simulink model "SalientPolePMSM"  (R2020b)
settings: Solver=VariableStepAuto  StartTime=0  StopTime=1  MaxStep=1e-4  RelTol=1e-4
values from neighbouring files (symbols this model uses):
  Bgain = 1    [DataSalientPolePMSM-DESKTOP-IINSHMA.m]    (also in DataSalientPolePMSM.m)
  Gcc_1ord = 1/(s/bandwidth(Gcc) + 1)    [DataSalientPolePMSM-DESKTOP-IINSHMA.m]    (also in DataSalientPolePMSM.m)
  lamdVec = mot.Ld*idVec+mot.lammg    [DataSalientPolePMSM-DESKTOP-IINSHMA.m]    (also in DataSalientPolePMSM.m)
  lamqVec = mot.Lq*iqVec    [DataSalientPolePMSM-DESKTOP-IINSHMA.m]    (also in DataSalientPolePMSM.m)
  TAB0_abc = Tabc_AB0^-1    [DataSalientPolePMSM-DESKTOP-IINSHMA.m]    (also in DataSalientPolePMSM.m)
  Tabc_AB0 = 2/3.*[     1       -1/2       -1/2 ... (first row only)    [DataSalientPolePMSM-DESKTOP-IINSHMA.m]    (also in DataSalientPolePMSM.m)
  Talphabeta_abc = Tabc_alphabeta^(-1)    [DataSalientPolePMSM-DESKTOP-IINSHMA.m]    (also in DataSalientPolePMSM.m)
undefined symbols (not defined in the file or in its folder): DiscIntNeverNeededParam, dqpll, inv, kid, kpd, magnitude, meas, mot, Obs, PI, stconv
libraries: simulink x53, pid_lib x3, powerlib x2, eeBldcCommutationLogic x1, electricdrivelib x1
(part 6 of 7)

== system SalientPolePMSM/FOC2/INVERTER2/INVERTER power driver ==
  note: INVERTER:
      | (-Ubus/2  :  +Ubus/2)
  note: INPUTS:
  note: OUTPUTS:
  note: solo Tpwm/2 perchè
      | controllo tempo discreto
  duties : Inport
  uBus : Inport  Port=2
  iabc : Inport  Port=3
  Constant1 : Constant  Value=0.5
  Inverter non idealities : Subsystem  Commented=on
  Product : Product
  Subtract : Sum  Inputs=+-
  Transport Delay : TransportDelay  DelayTime=inv.Tpwm/2
  delay_aproximation : Subsystem  Commented=on
  uabc_n* : Outport
  uabc_n*nonideal : Outport  Port=2
  wires:
  iabc/1 -> Inverter non idealities/3(iabc)
  duties/1 -> Subtract/1
  Inverter non idealities/1(uabc_dist) -> uabc_n*nonideal/1
  Constant1/1 -> Subtract/2
  uBus/1 -> Inverter non idealities/2(uBus), Product/2
  Product/1 -> Inverter non idealities/1(uabc), Transport Delay/1  "uabc"
  Subtract/1 -> Product/1
  Transport Delay/1 -> uabc_n*/1

== system SalientPolePMSM/FOC2/INVERTER2/SVM algorithm ==
  note: INPUTS:
      | voltage references
      | Alpha Beta axes
  note: OUTPUT
  VABref : Inport  PortDimensions=2
  uBus : Inport  Port=2  PortDimensions=1
  Gain : Gain  Gain=1000
  MATLAB Function : MATLAB Function  Commented=on  TreatAsAtomicUnit=on  SystemSampleTime=inv.Ts
  MATLAB Function1 : MATLAB Function  TreatAsAtomicUnit=on  SystemSampleTime=inv.Ts
  MATLAB Function2 : MATLAB Function  TreatAsAtomicUnit=on  SystemSampleTime=inv.Ts
  MATLAB Function4 : MATLAB Function  Commented=on  TreatAsAtomicUnit=on  SystemSampleTime=inv.Ts
  Mux : Mux  Commented=on  Inputs=3
  Mux1 : Mux  Inputs=3
  Scope : Scope  Commented=on  NumInputPorts=3
  Scope1 : Scope  Commented=on  NumInputPorts=2
  Scope2 : Scope  NumInputPorts=2
  duties : Outport  PortDimensions=3
  wires:
  Mux/1 -> MATLAB Function/1(XYZ)
  MATLAB Function4/3(Z) -> Scope/3, Mux/3
  MATLAB Function4/2(Y) -> Scope/2, Mux/2
  MATLAB Function4/1(X) -> Scope/1, Mux/1
  MATLAB Function/2(duty) -> Scope1/1
  uBus/1 -> [UBUS]
  VABref/1 -> MATLAB Function4/1(VABref), Gain/1
  MATLAB Function/1(sector) -> Scope1/2
  MATLAB Function1/3(Z) -> Mux1/3
  MATLAB Function1/2(Y) -> Mux1/2
  MATLAB Function1/1(X) -> Mux1/1
  Gain/1 -> MATLAB Function1/1(VABref)
  Mux1/1 -> MATLAB Function2/1(XYZ)
  MATLAB Function2/2(duty) -> duties/1, Scope2/1
  MATLAB Function2/1(sector) -> Scope2/2

== system SalientPolePMSM/INVERTER/INVERTER power driver/Inverter non idealities ==
  note: Transport delay: it
      | simulate the PWM
      | delay
  note: This allows to calculate the distortion voltages
      | with respect to the star point of the motor.
      | In fact, the motor model is built considering the
      | star point of the motor! Each voltage distortion
      | has been calculated with respect to the central
      | point of the inverter.
  uabc : Inport  PortDimensions=3
  uBus : Inport  Port=2  PortDimensions=1
  iabc : Inport  Port=3  PortDimensions=3
  Add : Sum
  Add1 : Sum  Inputs=-++
  Add2 : Sum
  Add3 : Sum
  Add4 : Sum  Inputs=+-
  Constant : Constant  Value=0.5
  Constant1 : Constant  Value=inv.nid.Vdm
  Divide : Product  Inputs=*/
  Gain : Gain  Gain=2*inv.nid.Vdm
  Gain1 : Gain  Gain=inv.nid.Vcm
  Gain2 : Gain  Gain=inv.nid.ttot/inv.Ts
  Gain3 : Gain  Gain=-1/3
  Product : Product
  Sign : Signum
  Sum of Elements : Sum  Inputs=+
  Transport Delay : TransportDelay  DelayTime=inv.Tpwm/2
  uabc_dist : Outport  PortDimensions=3
  wires:
  Constant/1 -> Add/2
  uabc/1 -> Add4/1, Divide/1
  uBus/1 -> Divide/2, Gain2/1
  Divide/1 -> Add/1
  Add/1 -> Gain/1
  Gain/1 -> Add1/1
  Constant1/1 -> Add1/2
  Gain1/1 -> Add1/3
  Gain2/1 -> Product/2
  iabc/1 -> Sign/1
  Sign/1 -> Gain1/1, Product/1
  Add1/1 -> Add2/1
  Product/1 -> Add2/2  "u_dist_abc_n"
  Add2/1 -> Sum of Elements/1, Add3/1  "uabc_n_dist"
  Sum of Elements/1 -> Gain3/1
  Gain3/1 -> Add3/2  "u_on"
  Add3/1 -> Add4/2  "uabc_o_dist"
  Add4/1 -> Transport Delay/1
  Transport Delay/1 -> uabc_dist/1

== system SalientPolePMSM/INVERTER/INVERTER power driver/delay_aproximation ==
  uabc : Inport
  Demux2 : Demux  Outputs=3
  Mux : Mux  Inputs=3
  Transfer Fcn : TransferFcn  Denominator=[inv.tauD 1]
  Transfer Fcn1 : TransferFcn  Denominator=[inv.tauD 1]
  Transfer Fcn2 : TransferFcn  Denominator=[inv.tauD 1]
  uabc_n* : Outport
  wires:
  Demux2/3 -> Transfer Fcn2/1
  Transfer Fcn/1 -> Mux/1
  Transfer Fcn2/1 -> Mux/3
  Transfer Fcn1/1 -> Mux/2
  Demux2/1 -> Transfer Fcn/1
  Demux2/2 -> Transfer Fcn1/1
  uabc/1 -> Demux2/1
  Mux/1 -> uabc_n*/1

== system SalientPolePMSM/Synchronous motor1/electrical equations/Clarke + Park 2 ==
  note: INPUTS
  note: OUTPUT
  abc : Inport
  thme : Inport  Port=2
  Add2 : Sum
  Add3 : Sum  Inputs=-+
  Cos2 : Trigonometry  Operator=cos
  Demux1 : Demux  Outputs=3
  Demux2 : Demux  Outputs=3
  Gain1 : Gain  Gain=Tabc_AB0  Multiplication=Matrix(K*u) (u vector)
  Gain10 : Gain  Gain=-1/sqrt(3)
  Gain9 : Gain  Gain=2
  Mux1 : Mux  Inputs=2
  Mux2 : Mux  Inputs=3
  Product{,1..3} (4 alike) : Product
  Scope : Scope  NumInputPorts=2
  Sin2 : Trigonometry
  Sum5 : Sum  Inputs=++|
  Terminator : Terminator
  dq : Outport
  U_A : Outport  Port=2
  U_B : Outport  Port=3
  wires:
  Demux2/3 -> Terminator/1
  Product/1 -> Add2/1
  Product1/1 -> Add2/2
  Cos2/1 -> Product/2, Product3/1
  Demux2/1 -> [U_A], Product3/2, Product1/1
  thme/1 -> Cos2/1, Sin2/1
  Product3/1 -> Add3/2
  Product2/1 -> Add3/1
  Demux2/2 -> [U_B], Product2/1, Product/1
  Sin2/1 -> Product2/2, Product1/2
  Mux1/1 -> dq/1
  Add3/1 -> Mux1/2
  Add2/1 -> Mux1/1
  Sum5/1 -> Gain10/1
  Gain9/1 -> Sum5/2
  Demux1/2 -> Gain9/1
  Demux1/3 -> Mux2/3
  Demux1/1 -> Mux2/1, Sum5/1
  Gain10/1 -> Mux2/2
  abc/1 -> Gain1/1, Demux1/1
  Gain1/1 -> Scope/1, Demux2/1
  [U_A] -> U_A/1
  [U_B] -> U_B/1

== system SalientPolePMSM/Synchronous motor1/electrical equations/Clarke + Park 3 ==
  note: OUTPUT
  note: INPUTS
  abc : Inport
  thme : Inport  Port=2
  Add2 : Sum
  Add3 : Sum  Inputs=-+
  Cos2 : Trigonometry  Operator=cos
  Demux2 : Demux  Outputs=3
  Gain : Gain  Gain=Tabc_AB0  Multiplication=Matrix(K*u) (u vector)
  Mux1 : Mux  Inputs=2
  Product{,1..3} (4 alike) : Product
  Sin2 : Trigonometry
  Terminator : Terminator
  dq : Outport
  wires:
  Mux1/1 -> dq/1
  Sin2/1 -> Product1/2, Product2/2
  Demux2/2 -> Product3/2, Product1/1
  Product2/1 -> Add3/1
  Product3/1 -> Add3/2
  thme/1 -> Sin2/1, Cos2/1
  Demux2/1 -> Product2/1, Product/1
  Cos2/1 -> Product3/1, Product/2
  Product1/1 -> Add2/2
  Add3/1 -> Mux1/2
  Add2/1 -> Mux1/1
  Product/1 -> Add2/1
  Gain/1 -> Demux2/1  "AB0"
  Demux2/3 -> Terminator/1
  abc/1 -> Gain/1

== system SalientPolePMSM/Synchronous motor1/electrical equations/Subsystem2 ==
  note: INPUTS
  note: OUTPUT
  thme : Inport
  abc : Inport  Port=2
  Add2 : Sum
  Add3 : Sum  Inputs=-+
  Cos2 : Trigonometry  Operator=cos
  Demux2 : Demux  Outputs=3
  Demux3 : Demux  Outputs=3
  Gain : Gain  Gain=Tabc_AB0  Multiplication=Matrix(K*u) (u vector)
  Gain2 : Gain  Gain=2
  Gain3 : Gain  Gain=-1/sqrt(3)
  Mux1 : Mux  Inputs=2
  Mux2 : Mux  Inputs=3
  Product{,1..3,5} (5 alike) : Product
  Sin2 : Trigonometry
  Terminator : Terminator
  qd : Outport
  wires:
  Demux2/3 -> Terminator/1
  Product/1 -> Add2/1
  Product1/1 -> Add2/2
  Cos2/1 -> Product/2, Product3/1
  Demux2/1 -> Product1/1, Product3/2
  thme/1 -> Cos2/1, Sin2/1
  Product3/1 -> Add3/2
  Product2/1 -> Add3/1
  Demux2/2 -> Product2/1, Product/1
  Sin2/1 -> Product2/2, Product1/2
  Mux1/1 -> qd/1
  Mux2/1 -> ?  "AB0"
  Gain2/1 -> Product5/2
  ? -> Demux3/1
  Demux3/1 -> Mux2/1, Product5/1
  Product5/1 -> Gain3/1
  Demux3/2 -> Gain2/1
  Demux3/3 -> Mux2/3
  Gain3/1 -> Mux2/2
  abc/1 -> Gain/1
  Gain/1 -> Demux2/1
  Add2/1 -> Mux1/1
  Add3/1 -> Mux1/2

== system SalientPolePMSM/Synchronous motor1/electrical equations/Subsystem4 ==
  note: INPUTS
  note: OUTPUT
  thme : Inport
  abc : Inport  Port=2
  Add2 : Sum
  Add3 : Sum  Inputs=-+
  Cos2 : Trigonometry  Operator=cos
  Demux1 : Demux  Outputs=3
  Demux2 : Demux  Outputs=3
  Gain : Gain  Gain=2
  Gain1 : Gain  Gain=-1/sqrt(3)
  Mux : Mux  Inputs=3
  Mux1 : Mux  Inputs=2
  Product{,1..4} (5 alike) : Product
  Sin2 : Trigonometry
  Terminator : Terminator
  dq : Outport
  wires:
  Demux1/3 -> Mux/3
  Gain1/1 -> Mux/2
  Product4/1 -> Gain1/1
  Gain/1 -> Product4/2
  Demux1/2 -> Gain/1
  Demux1/1 -> Mux/1, Product4/1
  abc/1 -> Demux1/1
  Demux2/3 -> Terminator/1
  Mux/1 -> Demux2/1  "AB0"
  Product/1 -> Add2/1
  Add2/1 -> Mux1/1
  Add3/1 -> Mux1/2
  Product1/1 -> Add2/2
  Cos2/1 -> Product/2, Product3/1
  Demux2/1 -> Product1/1, Product3/2
  thme/1 -> Cos2/1, Sin2/1
  Product3/1 -> Add3/2
  Product2/1 -> Add3/1
  Demux2/2 -> Product2/1, Product/1
  Sin2/1 -> Product2/2, Product1/2
  Mux1/1 -> dq/1

== system SalientPolePMSM/Synchronous motor2/electrical equations/Subsystem1 ==
  note: OUTPUT
  note: INPUTS
  abc : Inport
  thme : Inport  Port=2
  Add2 : Sum
  Add3 : Sum  Inputs=-+
  Cos2 : Trigonometry  Operator=cos
  Demux2 : Demux  Outputs=3
  Gain : Gain  Gain=Tabc_AB0  Multiplication=Matrix(K*u) (u vector)
  Mux1 : Mux  Inputs=2
  Product{,1..3} (4 alike) : Product
  Scope : Scope  NumInputPorts=2
  Sin2 : Trigonometry
  Terminator : Terminator
  dq : Outport
  wires:
  Mux1/1 -> dq/1
  Sin2/1 -> Product1/2, Product2/2
  Demux2/2 -> Product3/2, Product1/1
  Product2/1 -> Add3/1
  Product3/1 -> Add3/2
  thme/1 -> Sin2/1, Cos2/1
  Demux2/1 -> Product2/1, Product/1
  Cos2/1 -> Product3/1, Product/2
  Product1/1 -> Add2/2
  Add3/1 -> Mux1/2
  Add2/1 -> Mux1/1
  Product/1 -> Add2/1
  Gain/1 -> Scope/2, Demux2/1  "AB0"
  Demux2/3 -> Terminator/1
  abc/1 -> Scope/1, Gain/1

== system SalientPolePMSM/Synchronous motor3/electrical equations/Clarke + Park 2 ==
  note: INPUTS
  note: OUTPUT
  abc : Inport
  thme : Inport  Port=2
  Add2 : Sum
  Add3 : Sum  Inputs=-+
  Cos2 : Trigonometry  Operator=cos
  Demux1 : Demux  Outputs=3
  Demux2 : Demux  Outputs=3
  Gain1 : Gain  Gain=Tabc_AB0  Multiplication=Matrix(K*u) (u vector)
  Gain10 : Gain  Gain=-1/sqrt(3)
  Gain9 : Gain  Gain=2
  Mux1 : Mux  Inputs=2
  Mux2 : Mux  Inputs=3
  Product{,1..3} (4 alike) : Product
  Scope : Scope  NumInputPorts=2
  Sin2 : Trigonometry
  Sum5 : Sum  Inputs=++|
  Terminator : Terminator
  dq : Outport
  U_A : Outport  Port=2
  U_B : Outport  Port=3
  wires:
  Demux2/3 -> Terminator/1
  Product/1 -> Add2/1
  Product1/1 -> Add2/2
  Cos2/1 -> Product/2, Product3/1
  Demux2/1 -> [U_A], Product3/2, Product1/1
  thme/1 -> Cos2/1, Sin2/1
  Product3/1 -> Add3/2
  Product2/1 -> Add3/1
  Demux2/2 -> [U_B], Product2/1, Product/1
  Sin2/1 -> Product2/2, Product1/2
  Mux1/1 -> dq/1
  Add3/1 -> Mux1/2
  Add2/1 -> Mux1/1
  Sum5/1 -> Gain10/1
  Gain9/1 -> Sum5/2
  Demux1/2 -> Gain9/1
  Demux1/3 -> Mux2/3
  Demux1/1 -> Mux2/1, Sum5/1
  Gain10/1 -> Mux2/2
  abc/1 -> Gain1/1, Demux1/1
  Gain1/1 -> Scope/1, Demux2/1
  [U_A] -> U_A/1
  [U_B] -> U_B/1

== system SalientPolePMSM/Synchronous motor3/electrical equations/Clarke + Park 3 ==
  note: OUTPUT
  note: INPUTS
  abc : Inport
  thme : Inport  Port=2
  Add2 : Sum
  Add3 : Sum  Inputs=-+
  Cos2 : Trigonometry  Operator=cos
  Demux2 : Demux  Outputs=3
  Gain : Gain  Gain=Tabc_AB0  Multiplication=Matrix(K*u) (u vector)
  Mux1 : Mux  Inputs=2
  Product{,1..3} (4 alike) : Product
  Sin2 : Trigonometry
  Terminator : Terminator
  dq : Outport
  wires:
  Mux1/1 -> dq/1
  Sin2/1 -> Product1/2, Product2/2
  Demux2/2 -> Product3/2, Product1/1
  Product2/1 -> Add3/1
  Product3/1 -> Add3/2
  thme/1 -> Sin2/1, Cos2/1
  Demux2/1 -> Product2/1, Product/1
  Cos2/1 -> Product3/1, Product/2
  Product1/1 -> Add2/2
  Add3/1 -> Mux1/2
  Add2/1 -> Mux1/1
  Product/1 -> Add2/1
  Gain/1 -> Demux2/1  "AB0"
  Demux2/3 -> Terminator/1
  abc/1 -> Gain/1

== system SalientPolePMSM/Synchronous motor3/electrical equations/Subsystem2 ==
  note: INPUTS
  note: OUTPUT
  thme : Inport
  abc : Inport  Port=2
  Add2 : Sum
  Add3 : Sum  Inputs=-+
  Cos2 : Trigonometry  Operator=cos
  Demux2 : Demux  Outputs=3
  Demux3 : Demux  Outputs=3
  Gain : Gain  Gain=Tabc_AB0  Multiplication=Matrix(K*u) (u vector)
  Gain2 : Gain  Gain=2
  Gain3 : Gain  Gain=-1/sqrt(3)
  Mux1 : Mux  Inputs=2
  Mux2 : Mux  Inputs=3
  Product{,1..3,5} (5 alike) : Product
  Sin2 : Trigonometry
  Terminator : Terminator
  qd : Outport
  wires:
  Demux2/3 -> Terminator/1
  Product/1 -> Add2/1
  Product1/1 -> Add2/2
  Cos2/1 -> Product/2, Product3/1
  Demux2/1 -> Product1/1, Product3/2
  thme/1 -> Cos2/1, Sin2/1
  Product3/1 -> Add3/2
  Product2/1 -> Add3/1
  Demux2/2 -> Product2/1, Product/1
  Sin2/1 -> Product2/2, Product1/2
  Mux1/1 -> qd/1
  Mux2/1 -> ?  "AB0"
  Gain2/1 -> Product5/2
  ? -> Demux3/1
  Demux3/1 -> Mux2/1, Product5/1
  Product5/1 -> Gain3/1
  Demux3/2 -> Gain2/1
  Demux3/3 -> Mux2/3
  Gain3/1 -> Mux2/2
  abc/1 -> Gain/1
  Gain/1 -> Demux2/1
  Add2/1 -> Mux1/1
  Add3/1 -> Mux1/2

== system SalientPolePMSM/Synchronous motor3/electrical equations/Subsystem4 ==
  note: INPUTS
  note: OUTPUT
  thme : Inport
  abc : Inport  Port=2
  Add2 : Sum
  Add3 : Sum  Inputs=-+
  Cos2 : Trigonometry  Operator=cos
  Demux1 : Demux  Outputs=3
  Demux2 : Demux  Outputs=3
  Gain : Gain  Gain=2
  Gain1 : Gain  Gain=-1/sqrt(3)
  Mux : Mux  Inputs=3
  Mux1 : Mux  Inputs=2
  Product{,1..4} (5 alike) : Product
  Sin2 : Trigonometry
  Terminator : Terminator
  dq : Outport
  wires:
  Demux1/3 -> Mux/3
  Gain1/1 -> Mux/2
  Product4/1 -> Gain1/1
  Gain/1 -> Product4/2
  Demux1/2 -> Gain/1
  Demux1/1 -> Mux/1, Product4/1
  abc/1 -> Demux1/1
  Demux2/3 -> Terminator/1
  Mux/1 -> Demux2/1  "AB0"
  Product/1 -> Add2/1
  Add2/1 -> Mux1/1
  Add3/1 -> Mux1/2
  Product1/1 -> Add2/2
  Cos2/1 -> Product/2, Product3/1
  Demux2/1 -> Product1/1, Product3/2
  thme/1 -> Cos2/1, Sin2/1
  Product3/1 -> Add3/2
  Product2/1 -> Add3/1
  Demux2/2 -> Product2/1, Product/1
  Sin2/1 -> Product2/2, Product1/2
  Mux1/1 -> dq/1

== system SalientPolePMSM/FOC1/INVERTER1/INVERTER power driver/Inverter non idealities ==
  note: This allows to calculate the distortion voltages
      | with respect to the star point of the motor.
      | In fact, the motor model is built considering the
      | star point of the motor! Each voltage distortion
      | has been calculated with respect to the central
      | point of the inverter.
  note: Transport delay: it
      | simulate the PWM
      | delay
  uabc : Inport  PortDimensions=3
  uBus : Inport  Port=2  PortDimensions=1
  iabc : Inport  Port=3  PortDimensions=3
  Add : Sum
  Add1 : Sum  Inputs=-++
  Add2 : Sum
  Add3 : Sum
  Add4 : Sum  Inputs=+-
  Constant : Constant  Value=0.5
  Constant1 : Constant  Value=inv.nid.Vdm
  Divide : Product  Inputs=*/
  Gain : Gain  Gain=2*inv.nid.Vdm
  Gain1 : Gain  Gain=inv.nid.Vcm
  Gain2 : Gain  Gain=inv.nid.ttot/inv.Ts
  Gain3 : Gain  Gain=-1/3
  Product : Product
  Sign : Signum
  Sum of Elements : Sum  Inputs=+
  Transport Delay : TransportDelay  DelayTime=inv.Tpwm/2
  uabc_dist : Outport  PortDimensions=3
  wires:
  Transport Delay/1 -> uabc_dist/1
  Add4/1 -> Transport Delay/1
  Add3/1 -> Add4/2  "uabc_o_dist"
  Gain3/1 -> Add3/2  "u_on"
  Sum of Elements/1 -> Gain3/1
  Add2/1 -> Add3/1, Sum of Elements/1  "uabc_n_dist"
  Product/1 -> Add2/2  "u_dist_abc_n"
  Add1/1 -> Add2/1
  Sign/1 -> Product/1, Gain1/1
  iabc/1 -> Sign/1
  Gain2/1 -> Product/2
  Gain1/1 -> Add1/3
  Constant1/1 -> Add1/2
  Gain/1 -> Add1/1
  Add/1 -> Gain/1
  Divide/1 -> Add/1
  uBus/1 -> Gain2/1, Divide/2
  uabc/1 -> Divide/1, Add4/1
  Constant/1 -> Add/2

== system SalientPolePMSM/FOC1/INVERTER1/INVERTER power driver/delay_aproximation ==
  uabc : Inport
  Demux2 : Demux  Outputs=3
  Mux : Mux  Inputs=3
  Transfer Fcn : TransferFcn  Denominator=[inv.tauD 1]
  Transfer Fcn1 : TransferFcn  Denominator=[inv.tauD 1]
  Transfer Fcn2 : TransferFcn  Denominator=[inv.tauD 1]
  uabc_n* : Outport
  wires:
  Mux/1 -> uabc_n*/1
  uabc/1 -> Demux2/1
  Demux2/2 -> Transfer Fcn1/1
  Demux2/1 -> Transfer Fcn/1
  Transfer Fcn1/1 -> Mux/2
  Transfer Fcn2/1 -> Mux/3
  Transfer Fcn/1 -> Mux/1
  Demux2/3 -> Transfer Fcn2/1

== system SalientPolePMSM/FOC1/INVERTER2/INVERTER power driver/Inverter non idealities ==
  note: This allows to calculate the distortion voltages
      | with respect to the star point of the motor.
      | In fact, the motor model is built considering the
      | star point of the motor! Each voltage distortion
      | has been calculated with respect to the central
      | point of the inverter.
  note: Transport delay: it
      | simulate the PWM
      | delay
  uabc : Inport  PortDimensions=3
  uBus : Inport  Port=2  PortDimensions=1
  iabc : Inport  Port=3  PortDimensions=3
  Add : Sum
  Add1 : Sum  Inputs=-++
  Add2 : Sum
  Add3 : Sum
  Add4 : Sum  Inputs=+-
  Constant : Constant  Value=0.5
  Constant1 : Constant  Value=inv.nid.Vdm
  Divide : Product  Inputs=*/
  Gain : Gain  Gain=2*inv.nid.Vdm
  Gain1 : Gain  Gain=inv.nid.Vcm
  Gain2 : Gain  Gain=inv.nid.ttot/inv.Ts
  Gain3 : Gain  Gain=-1/3
  Product : Product
  Sign : Signum
  Sum of Elements : Sum  Inputs=+
  Transport Delay : TransportDelay  DelayTime=inv.Tpwm/2
  uabc_dist : Outport  PortDimensions=3
  wires:
  Transport Delay/1 -> uabc_dist/1
  Add4/1 -> Transport Delay/1
  Add3/1 -> Add4/2  "uabc_o_dist"
  Gain3/1 -> Add3/2  "u_on"
  Sum of Elements/1 -> Gain3/1
  Add2/1 -> Add3/1, Sum of Elements/1  "uabc_n_dist"
  Product/1 -> Add2/2  "u_dist_abc_n"
  Add1/1 -> Add2/1
  Sign/1 -> Product/1, Gain1/1
  iabc/1 -> Sign/1
  Gain2/1 -> Product/2
  Gain1/1 -> Add1/3
  Constant1/1 -> Add1/2
  Gain/1 -> Add1/1
  Add/1 -> Gain/1
  Divide/1 -> Add/1
  uBus/1 -> Gain2/1, Divide/2
  uabc/1 -> Divide/1, Add4/1
  Constant/1 -> Add/2

== system SalientPolePMSM/FOC1/INVERTER2/INVERTER power driver/delay_aproximation ==
  uabc : Inport
  Demux2 : Demux  Outputs=3
  Mux : Mux  Inputs=3
  Transfer Fcn : TransferFcn  Denominator=[inv.tauD 1]
  Transfer Fcn1 : TransferFcn  Denominator=[inv.tauD 1]
  Transfer Fcn2 : TransferFcn  Denominator=[inv.tauD 1]
  uabc_n* : Outport
  wires:
  Mux/1 -> uabc_n*/1
  uabc/1 -> Demux2/1
  Demux2/2 -> Transfer Fcn1/1
  Demux2/1 -> Transfer Fcn/1
  Transfer Fcn1/1 -> Mux/2
  Transfer Fcn2/1 -> Mux/3
  Transfer Fcn/1 -> Mux/1
  Demux2/3 -> Transfer Fcn2/1

== system SalientPolePMSM/FOC2/INVERTER1/INVERTER power driver/Inverter non idealities ==
  note: This allows to calculate the distortion voltages
      | with respect to the star point of the motor.
      | In fact, the motor model is built considering the
      | star point of the motor! Each voltage distortion
      | has been calculated with respect to the central
      | point of the inverter.
  note: Transport delay: it
      | simulate the PWM
      | delay
  uabc : Inport  PortDimensions=3
  uBus : Inport  Port=2  PortDimensions=1
  iabc : Inport  Port=3  PortDimensions=3
  Add : Sum
  Add1 : Sum  Inputs=-++
  Add2 : Sum
  Add3 : Sum
  Add4 : Sum  Inputs=+-
  Constant : Constant  Value=0.5
  Constant1 : Constant  Value=inv.nid.Vdm
  Divide : Product  Inputs=*/
  Gain : Gain  Gain=2*inv.nid.Vdm
  Gain1 : Gain  Gain=inv.nid.Vcm
  Gain2 : Gain  Gain=inv.nid.ttot/inv.Ts
  Gain3 : Gain  Gain=-1/3
  Product : Product
  Sign : Signum
  Sum of Elements : Sum  Inputs=+
  Transport Delay : TransportDelay  DelayTime=inv.Tpwm/2
  uabc_dist : Outport  PortDimensions=3
  wires:
  Transport Delay/1 -> uabc_dist/1
  Add4/1 -> Transport Delay/1
  Add3/1 -> Add4/2  "uabc_o_dist"
  Gain3/1 -> Add3/2  "u_on"
  Sum of Elements/1 -> Gain3/1
  Add2/1 -> Add3/1, Sum of Elements/1  "uabc_n_dist"
  Product/1 -> Add2/2  "u_dist_abc_n"
  Add1/1 -> Add2/1
  Sign/1 -> Product/1, Gain1/1
  iabc/1 -> Sign/1
  Gain2/1 -> Product/2
  Gain1/1 -> Add1/3
  Constant1/1 -> Add1/2
  Gain/1 -> Add1/1
  Add/1 -> Gain/1
  Divide/1 -> Add/1
  uBus/1 -> Gain2/1, Divide/2
  uabc/1 -> Divide/1, Add4/1
  Constant/1 -> Add/2

== system SalientPolePMSM/FOC2/INVERTER1/INVERTER power driver/delay_aproximation ==
  uabc : Inport
  Demux2 : Demux  Outputs=3
  Mux : Mux  Inputs=3
  Transfer Fcn : TransferFcn  Denominator=[inv.tauD 1]
  Transfer Fcn1 : TransferFcn  Denominator=[inv.tauD 1]
  Transfer Fcn2 : TransferFcn  Denominator=[inv.tauD 1]
  uabc_n* : Outport
  wires:
  Mux/1 -> uabc_n*/1
  uabc/1 -> Demux2/1
  Demux2/2 -> Transfer Fcn1/1
  Demux2/1 -> Transfer Fcn/1
  Transfer Fcn1/1 -> Mux/2
  Transfer Fcn2/1 -> Mux/3
  Transfer Fcn/1 -> Mux/1
  Demux2/3 -> Transfer Fcn2/1

== system SalientPolePMSM/FOC2/INVERTER2/INVERTER power driver/Inverter non idealities ==
  note: This allows to calculate the distortion voltages
      | with respect to the star point of the motor.
      | In fact, the motor model is built considering the
      | star point of the motor! Each voltage distortion
      | has been calculated with respect to the central
      | point of the inverter.
  note: Transport delay: it
      | simulate the PWM
      | delay
  uabc : Inport  PortDimensions=3
  uBus : Inport  Port=2  PortDimensions=1
  iabc : Inport  Port=3  PortDimensions=3
  Add : Sum
  Add1 : Sum  Inputs=-++
  Add2 : Sum
  Add3 : Sum
  Add4 : Sum  Inputs=+-
  Constant : Constant  Value=0.5
  Constant1 : Constant  Value=inv.nid.Vdm
  Divide : Product  Inputs=*/
  Gain : Gain  Gain=2*inv.nid.Vdm
  Gain1 : Gain  Gain=inv.nid.Vcm
  Gain2 : Gain  Gain=inv.nid.ttot/inv.Ts
  Gain3 : Gain  Gain=-1/3
  Product : Product
  Sign : Signum
  Sum of Elements : Sum  Inputs=+
  Transport Delay : TransportDelay  DelayTime=inv.Tpwm/2
  uabc_dist : Outport  PortDimensions=3
  wires:
  Transport Delay/1 -> uabc_dist/1
  Add4/1 -> Transport Delay/1
  Add3/1 -> Add4/2  "uabc_o_dist"
  Gain3/1 -> Add3/2  "u_on"
  Sum of Elements/1 -> Gain3/1
  Add2/1 -> Add3/1, Sum of Elements/1  "uabc_n_dist"
  Product/1 -> Add2/2  "u_dist_abc_n"
  Add1/1 -> Add2/1
  Sign/1 -> Product/1, Gain1/1
  iabc/1 -> Sign/1
  Gain2/1 -> Product/2
  Gain1/1 -> Add1/3
  Constant1/1 -> Add1/2
  Gain/1 -> Add1/1
  Add/1 -> Gain/1
  Divide/1 -> Add/1
  uBus/1 -> Gain2/1, Divide/2
  uabc/1 -> Divide/1, Add4/1
  Constant/1 -> Add/2

== system SalientPolePMSM/FOC2/INVERTER2/INVERTER power driver/delay_aproximation ==
  uabc : Inport
  Demux2 : Demux  Outputs=3
  Mux : Mux  Inputs=3
  Transfer Fcn : TransferFcn  Denominator=[inv.tauD 1]
  Transfer Fcn1 : TransferFcn  Denominator=[inv.tauD 1]
  Transfer Fcn2 : TransferFcn  Denominator=[inv.tauD 1]
  uabc_n* : Outport
  wires:
  Mux/1 -> uabc_n*/1
  uabc/1 -> Demux2/1
  Demux2/2 -> Transfer Fcn1/1
  Demux2/1 -> Transfer Fcn/1
  Transfer Fcn1/1 -> Mux/2
  Transfer Fcn2/1 -> Mux/3
  Transfer Fcn/1 -> Mux/1
  Demux2/3 -> Transfer Fcn2/1

== matlab function SalientPolePMSM/SENSORLESS ==
  data: iabc input; thme_est output; uabc input; ON_approx input; wme_est output; dqpll parameter; data input
function [thme_est,wme_est] = dqPLL_Sensorless(iabc, uabc, ON_approx, dqpll, data)

% sensorless algorithm based on dq-PLL loop

persistent Xd_1 Xq_1 thme_est_1 wme_est_1 ui_1 Dth_1
if isempty(Xd_1)
    Xd_1 = [0 0]';
    Xq_1 = [0 0]';
    thme_est_1 = 0;
    wme_est_1 = 0;
end
if isempty(ui_1)
    ui_1 = 0;
    Dth_1 = 0;
end

% compute abc->dq transformation
iAB0 = dqpll.Tabc_AB0*iabc;
idq = zeros(1,2);
idq(1) = iAB0(1)*cos(thme_est_1)+iAB0(2)*sin(thme_est_1);
idq(2) = -iAB0(1)*sin(thme_est_1)+iAB0(2)*cos(thme_est_1);

uAB0 = dqpll.Tabc_AB0*uabc;
udq = zeros(1,2);
udq(1) = uAB0(1)*cos(thme_est_1)+uAB0(2)*sin(thme_est_1);
udq(2) = -uAB0(1)*sin(thme_est_1)+uAB0(2)*cos(thme_est_1);

% DECOUPLING for ud and uq
udq(1) = udq(1) + wme_est_1*idq(2)*dqpll.Lq;
udq(2) = udq(2) - wme_est_1*idq(1)*dqpll.Lq;

% ESTIMATOR of ed and eq
Xd = dqpll.est.F1*Xd_1 + dqpll.est.G1*[udq(1) idq(1)]';
Xq = dqpll.est.F1*Xq_1 + dqpll.est.G1*[udq(2) idq(2)]';
ed = dqpll.est.H1*Xd;
eq = dqpll.est.H1*Xq;

% atan calculation
if ON_approx == 0
    Dth = atan2(-ed,eq);
else
    if abs(wme_est_1)<dqpll.minw
        w = dqpll.minw;
    else
        w = wme_est_1;
    end
    Eex = w*((dqpll.Ld-dqpll.Lq)*idq(1)+dqpll.lammg);
    Dth = -ed/Eex;
end

% PI loop
up = Dth*dqpll.PI.kp;
ui = ui_1 + Dth_1*dqpll.Ts;
wme = up + ui*dqpll.PI.ki;

% calculation of thme with EULER INTEGRATION
thme_est = thme_est_1 + dqpll.Ts*wme;

% Low Pass Filter for wme_est
wme_est = dqpll.lpf.alpha*wme + (1-dqpll.lpf.alpha)*wme_est_1;

% update variables
thme_est_1 = thme_est;
wme_est_1 = wme_est;
ui_1 = ui;
Dth_1 = Dth;
Xd_1 = Xd;
Xq_1 = Xq;

== matlab function SalientPolePMSM/SENSORLESS ALGORITHM/atanApprox ==
  data: id input; ed input; thme output; wme_est input; dqpll parameter
function thme = approx(id, ed, wme_est, dqpll)
if abs(wme_est)<dqpll.minw
    wme_est = dqpll.minw;
end
Eex = wme_est*((dqpll.Ld-dqpll.Lq)*id+dqpll.lammg);
thme = -ed/Eex;

== matlab function SalientPolePMSM/SENSORLESS ALGORITHM/atan ==
  data: ed input; thme output; eq input
function thme = atan(ed,eq)

thme = atan2(-ed,eq);

== matlab function SalientPolePMSM/MATLAB Function ==
  data: OffMtpa input; id output; i_ref input; iq output; mtpa parameter
function [id, iq]= MTPA(OffMtpa, i_ref, mtpa)
% Maximum Torque Per Ampere
if (mtpa.Ld==mtpa.Lq)||OffMtpa   % MTPA for PMSM
    id = 0;
    iq = i_ref;
else  % MTPA for IPMSM motor, or Salient Pole PMSM
    id = (mtpa.lammg-sqrt(mtpa.lammg^2+8*(mtpa.Ld-mtpa.Lq)^2*i_ref^2)/(-4*(mtpa.Ld-mtpa.Lq)));
    if i_ref>0
        iq = sqrt(i_ref^2-id^2);
        
    else
        iq = -sqrt(i_ref^2-id^2);
    end    
end

== matlab function SalientPolePMSM/MATLAB Function1 ==
  data: th input; thMod output
function thMod = ModulAxis(th)
% th[rad]-> 0<thMod<2*pi
n = abs(th/(2*pi));
if n>1
    if th>0
        thMod = th-floor(n)*2*pi;
    else
        thMod = th+floor(n)*2*pi;
    end
else
    thMod = th;
end

== matlab function SalientPolePMSM/MATLAB Function2 ==
  data: th input; thMod output
function thMod = ModulAxis(th)
% th[rad]-> 0<thMod<2*pi
n = abs(th/(2*pi));
if n>1
    if th>0
        thMod = th-floor(n)*2*pi;
    else
        thMod = th+floor(n)*2*pi;
    end
else
    thMod = th;
end

== matlab function SalientPolePMSM/FOC1/Circle Limitation/MATLAB Function ==
  data: u_d input; new_d output; u_q input; new_q output
function  [new_d, new_q] = Circle_limit(u_d,u_q)
if(u_d < 0)
    sign_d = -1;
else
    sign_d = 1;
end
if(u_q < 0)
    sign_q = -1;
else
    sign_q = 1;
end
    
sq_d = u_d*u_d;
sq_q = u_q*u_q;
maxModule = 31783; %PWM MAX MODELULATION 97%
sq_sum = sq_d + sq_q;
sq_limit = maxModule*maxModule;
MaxVd = (maxModule *950/1000);
sq_limit_d = MaxVd*MaxVd;
new_d = sqrt(sq_d) * sign_d;
new_q = sqrt(sq_q) * sign_q;

if(sq_sum > sq_limit)
    if (sq_d <= sq_limit_d)
        sq_tmp = sq_limit - sq_d;
        new_q = sqrt(sq_tmp);

        if (sqrt(sq_q) <= 0)
            new_q = -new_q;
        end
        new_d = sqrt(sq_d);
    else
        new_d = sq_limit_d;
        if( sqrt(sq_d) < 0)
            new_d = -new_d;
        end
        sq_tmp = sq_limit - sq_limit_d;
        new_q = sqrt(sq_tmp);
        
        if(sqrt(sq_q) < 0)
            new_q = - new_q;
        end
    end
end  

end

== matlab function SalientPolePMSM/DT SENSORLESS ALGORITHM DQ/MATLAB Function1 ==
  data: u input; y output
function y = fcn(u)

if(u < 0)
    y = u * -1;
else
    y = u;
end

== matlab function SalientPolePMSM/FOC1/INVERTER2/SVM algorithm/MATLAB Function1 ==
  data: VABref input; X output; Y output; Z output
function [X,Y,Z] = AB2XYZ(VABref)
% this function find the sector in the SVM where uABref is

PWM_period = 5250;
Valpha = VABref(1);
Vbeta = VABref(2);

Ualpha = Valpha * sqrt(3) * PWM_period * 2;
Ubeta = -(Vbeta * PWM_period)* 2;

X = Ubeta;
Y = (Ubeta + Ualpha)/2;
Z = (Ubeta - Ualpha) / 2;
end

== matlab function SalientPolePMSM/FOC1/INVERTER2/SVM algorithm/MATLAB Function2 ==
  data: XYZ input; sector output; duty output
function [sector,duty] = sector_identifier(XYZ)
% this function find the sector in the SVM where uABref is
PWMperiod = 5250;

X = XYZ(1);
Y = XYZ(2);
Z = XYZ(3);

TimePhA = 0;
TimePhB = 0; 
TimePhC = 0;

if(Y < 0) 
    if(Z < 0) 
        sector = 5;
        TimePhA = (PWMperiod/4) + (Y - Z)/262144;
        TimePhB = TimePhA + Z/131072;
        TimePhC = TimePhA - Y/131072;
    else
        if( X <= 0)
            sector = 4;
            TimePhA = (PWMperiod/4) + (X - Z)/262144;
            TimePhB = TimePhA + Z/131072;
            TimePhC = TimePhB - X/131072;
        else
            sector = 3;
            TimePhA = (PWMperiod/4) + (Y - X) /262144;
            TimePhC = TimePhA - Y/131072;
            TimePhB = TimePhC + X/131072;
        end
    end
else
    if(Z>=0)
        sector = 2;
        TimePhA = (PWMperiod/4) + (Y - Z)/262144;
        TimePhB = TimePhA + Z/131072;
        TimePhC = TimePhA - Y/131072;
    else
        if (X<=0)
            sector = 6;
            TimePhA = (PWMperiod/4) + (Y - X) /262144;
            TimePhC = TimePhA - Y/131072;
            TimePhB = TimePhC + X/131072;
        else
            sector = 1;
            TimePhA = (PWMperiod/4) + (X - Z)/262144;
            TimePhB = TimePhA + Z/131072;
            TimePhC = TimePhB - X/131072;
        end
    end
end

duty = [2*TimePhA/5250, 2*TimePhB/5250, 2*TimePhC/5250];
end

== matlab function SalientPolePMSM/FOC1/MATLAB Function ==
  data: sens input; vdout output size=1 [0..3000]; v input; speed input; vqout output size=1 [0..3000]
function [vdout,vqout] = startup(sens,v,speed)
persistent vq;
if isempty(vq)
    vq =0;
end
if(sens == 0)
    vq = vq + 0.00001;
    vqout = 0.5;
    vdout = 0;
else
    vqout = v(2);
    vdout = v(1);
end

if(speed > 60*5)
    sens = 0;
end

== matlab function SalientPolePMSM/Synchronous motor3/SPM Motor/MATLAB Function ==
  data: u input; B output
function B = fcn(u)
if( u>199)
    B = 0.0123;
else
    B = 0.006;
end

== matlab function SalientPolePMSM/Synchronous motor3/electrical equations/MATLAB Function ==
  data: i input; y output; Id_LUT parameter
function y = Vd_error(i,Id_LUT)
y = -0.1802*exp(-1.796*i)+0.1717;

== matlab function SalientPolePMSM/Fuzzy PI1/  ==
  data: err input; isMember_P output; isNotMember_P output; isMember_I output; isNotMember_I output; rule parameter
function [isMember_P, isNotMember_P,isMember_I, isNotMember_I] = Fuzzification(err, rule)
    persistent err_acc
    if isempty(err_acc)
        err_acc =0;
    end
    %calculate accumulate error
    err_acc = err_acc + err*20; % I- part

    %fuzzification for proportional term
    isMember_P = 0;
    isNotMember_P = 0;
    
    isMember_I = 0;
    isNotMember_I = 0;
    
    if( err >= rule.P.LIMIT )
        in_set = 1.0;
    elseif( err <= -rule.P.LIMIT  )
         in_set = 0.0;
    else
         in_set = (err + rule.P.LIMIT ) /(rule.P.LIMIT + rule.P.LIMIT );
    end
         
    isMember_P    = in_set * rule.P.WEIGHT;
    isNotMember_P =  (1.0 - in_set) * rule.P.WEIGHT;
    
    %fuzzification for integral term
    if( err_acc >= rule.I.LIMIT )
        in_set = 1.0;
    elseif( err_acc <= -rule.I.LIMIT  )
         in_set = 0.0;
    else
         in_set = (err_acc + rule.I.LIMIT ) /(rule.I.LIMIT + rule.I.LIMIT );
    end
         
    isMember_I    = in_set * rule.I.WEIGHT;
    isNotMember_I =  (1.0 - in_set) * rule.I.WEIGHT;
end

% void   evaluate_support(
%     float variable, rule *pRule, float *isMember, float *isNotMember )
% {
%     float  in_set;
%     if       ( variable >= pRule->highlimit )
%         in_set = 1.0;
%     else if  ( variable <= pRule->lowlimit )
%         in_set = 0.0;
%     else
%         in_set = (variable - pRule->lowlimit) /
%                  (pRule->highlimit - pRule->lowlimit);
% }

== matlab function SalientPolePMSM/INVERTER/SVM algorithm/MATLAB Function1 ==
  data: UABref input; uABref_sat output; uBus input; satON output
function [uABref_sat, satON] = circle_sat(UABref, uBus)
%

den = UABref(1)^2 + UABref(2)^2;
num = uBus^2/3;

if den > num
    satON = 1;
    k = sqrt(num/den);
    uABref_sat = (k.*UABref);
else
   uABref_sat = UABref; 
   satON = 0;
end

== matlab function SalientPolePMSM/MATLAB Function3 ==
  data: OffMtpa input; id output; i_ref input; iq output; mtpa parameter
function [id, iq]= MTPA(OffMtpa, i_ref, mtpa)
% Maximum Torque Per Ampere
if (mtpa.Ld==mtpa.Lq)||OffMtpa   % MTPA for PMSM
    id = 0;
    iq = i_ref;
else  % MTPA for IPMSM motor, or Salient Pole PMSM
    id = (mtpa.lammg-sqrt(mtpa.lammg^2+8*(mtpa.Ld-mtpa.Lq)^2*i_ref^2)/(-4*(mtpa.Ld-mtpa.Lq)));
    if i_ref>0
        iq = sqrt(i_ref^2-id^2);
        
    else
        iq = -sqrt(i_ref^2-id^2);
    end    
end

== matlab function SalientPolePMSM/Fuzzy PI/  ==
  data: err input; isMember_P output; isNotMember_P output; isMember_I output; isNotMember_I output; rule parameter
function [isMember_P, isNotMember_P,isMember_I, isNotMember_I] = Fuzzification(err, rule)
    persistent err_acc
    if isempty(err_acc)
        err_acc =0;
    end
    %calculate accumulate error
    err_acc = err_acc + err; % I- part

    %fuzzification for proportional term
    isMember_P = 0;
    isNotMember_P = 0;
    
    isMember_I = 0;
    isNotMember_I = 0;
    
    if       ( err >= rule.P.LIMIT )
        in_set = 1.0;
    elseif  ( err <= -rule.P.LIMIT  )
         in_set = 0.0;
    else
         in_set = (err + rule.P.LIMIT ) /(rule.P.LIMIT + rule.P.LIMIT );
    end
         
    isMember_P    = in_set * rule.P.WEIGHT;
    isNotMember_P =  (1.0 - in_set) * rule.P.WEIGHT;
    
    %fuzzification for integral term
    if       ( err_acc >= rule.I.LIMIT )
        in_set = 1.0;
    elseif  ( err_acc <= -rule.I.LIMIT  )
         in_set = 0.0;
    else
         in_set = (err_acc + rule.I.LIMIT ) /(rule.I.LIMIT + rule.I.LIMIT );
    end
         
    isMember_I    = in_set * rule.I.WEIGHT;
    isNotMember_I =  (1.0 - in_set) * rule.I.WEIGHT;
end

% void   evaluate_support(
%     float variable, rule *pRule, float *isMember, float *isNotMember )
% {
%     float  in_set;
%     if       ( variable >= pRule->highlimit )
%         in_set = 1.0;
%     else if  ( variable <= pRule->lowlimit )
%         in_set = 0.0;
%     else
%         in_set = (variable - pRule->lowlimit) /
%                  (pRule->highlimit - pRule->lowlimit);
% }

== matlab function SalientPolePMSM/Fuzzy PI/   ==
  data: isMember_P input; isNotMember_P input; isMember output; isMember_I input; isNotMember_I input; isNotMember output
function [isMember, isNotMember] = Inference(isMember_P, isNotMember_P, isMember_I, isNotMember_I)
isMember = isMember_P + isMember_I;
isNotMember = isNotMember_P + isNotMember_I;
end

% float   compute_fuzzy_PID ( float  Err, float  AccumErr, float  Speed )
% {
%     float  isMember = 0.0;
%     float  isNotMember = 0.0;
%     evaluate_support( Err,      &P_rule, &isMember, &isNotMember );
%     evaluate_support( AccumErr, &I_rule, &isMember, &isNotMember );
%     evaluate_support( Speed,    &D_rule, &isMember, &isNotMember );
%     return  defuzzify( &O_rule, isMember, isNotMember );
% }

== matlab function SalientPolePMSM/Fuzzy PI/    ==
  data: isMember input; tau output; isNotMember input; rule parameter
function tau = Defuzification(isMember, isNotMember, rule)

tau = (isMember * rule.O.LIMIT) + (isNotMember * -rule.O.LIMIT);

%saturation output
if  (tau > rule.O.LIMIT)  
tau = rule.O.LIMIT;
end
if  (tau < -rule.O.LIMIT)   
tau = -rule.O.LIMIT;
end
end

% float  defuzzify( rule *pRule, float isMember, float isNotMember )
% {
%     float  output;
%     output = (isMember * pRule->highlimit) + (isNotMember * pRule->lowlimit);
%     if  (output>pRule->highlimit)  output=pRule->highlimit;
%     if  (output>pRule->lowlimit)   output=pRule->lowlimit;
%     return output;
% }

== matlab function SalientPolePMSM/FOC1/INVERTER1/SVM algorithm/MATLAB Function ==
  data: uABref input; sector output
function sector = sector_identifier(uABref)
% this function find the sector in the SVM where uABref is
ua = uABref(1);
ub = uABref(2);

if(ub > 0) 
    if(abs(ua) > abs(ub)/sqrt(3))
        if (ua > 0)
            sector=1;
        else
            sector=3;
        end
    else
        sector=2;
    end
else
    if(abs(ua) > abs(ub)/sqrt(3))
        if (ua > 0)
            sector=6;
        else 
            sector=4;
        end
    else
        sector=5;
    end
end

== matlab function SalientPolePMSM/Fuzzy PI/Rule base ==
  data: y output
function y = fcn()

y = 0;

== matlab function SalientPolePMSM/Discrete SS ALGORITHM1/atan ==
  data: ed input; thme output; eq input
function thme = atan(ed,eq)

thme = atan2(-ed,eq);

== matlab function SalientPolePMSM/Discrete SS ALGORITHM1/atanApprox ==
  data: id input; ed input; thme output; wme_est input; dqpll parameter
function thme = approx(id, ed, wme_est, dqpll)
if abs(wme_est)<dqpll.minw
    wme_est = dqpll.minw;
end
Eex = wme_est*((dqpll.Ld-dqpll.Lq)*id+dqpll.lammg);
thme = -ed/Eex;

== matlab function SalientPolePMSM/FOC1/INVERTER1/SVM algorithm/MATLAB Function1 ==
  data: UABref input; uABref_sat output; uBus input; satON output
function [uABref_sat, satON] = circle_sat(UABref, uBus)
%

den = UABref(1)^2 + UABref(2)^2;
num = uBus^2/3;

if den > num
    satON = 1;
    k = sqrt(num/den);
    uABref_sat = (k.*UABref);
else
   uABref_sat = UABref; 
   satON = 0;
end

== matlab function SalientPolePMSM/FOC1/INVERTER1/SVM algorithm/MATLAB Function2 ==
  data: sid input; Tm_m1_0 output; uABref input; uBus input; inv parameter
function Tm_m1_0 = application_time(sid, uABref, uBus, inv)
%this function calculate the application time Tm Tm+1 and T0

Tm_m1_0 = zeros(3,1);

    % PROBLEMA DI PASSAGGIO DELLA VARIABILE ALLA FUNZIONE

Tm_m1_0(1)=sqrt(3)/uBus*inv.Tpwm*(uABref(1)*inv.sector_LUT(sid,1)-uABref(2)*inv.sector_LUT(sid,2));
Tm_m1_0(2)=sqrt(3)/uBus*inv.Tpwm*(-uABref(1)*inv.sector_LUT(sid,3)+uABref(2)*inv.sector_LUT(sid,4));
Tm_m1_0(3)=inv.Tpwm-Tm_m1_0(1)-Tm_m1_0(2);

== matlab function SalientPolePMSM/INVERTER/SVM algorithm/MATLAB Function ==
  data: uABref input; sector output
function sector = sector_identifier(uABref)
% this function find the sector in the SVM where uABref is
ua = uABref(1);
ub = uABref(2);

if(ub > 0) 
    if(abs(ua) > abs(ub)/sqrt(3))
        if (ua > 0)
            sector=1;
        else
            sector=3;
        end
    else
        sector=2;
    end
else
    if(abs(ua) > abs(ub)/sqrt(3))
        if (ua > 0)
            sector=6;
        else 
            sector=4;
        end
    else
        sector=5;
    end
end

== matlab function SalientPolePMSM/FOC1/INVERTER1/SVM algorithm/MATLAB Function3 ==
  data: sid input; Tm_m1_0 input; uABref input; uAref_sat output; uBref_sat output; duties output; Tabc_AB0 parameter; inv parameter; satON output
function [uAref_sat, uBref_sat, duties, satON] = hexagonal_sat_sat(sid, Tm_m1_0, uABref, Tabc_AB0, inv)
%

% hexagonal saturation
if Tm_m1_0(3)<0
    satON = 1;
    k = inv.Tpwm/(Tm_m1_0(1)+Tm_m1_0(2));
    Tm_m1_0 = k.*Tm_m1_0;
    Tm_m1_0(3) = 0;
else
    satON = 0;
end

% duties calculation
duties = zeros(3,1);

switch sid
    case 1
        duties(1) = (Tm_m1_0(1)+Tm_m1_0(2)+Tm_m1_0(3)/2);
        duties(2) = (Tm_m1_0(2)+Tm_m1_0(3)/2);
        duties(3) = (Tm_m1_0(3)/2);
    case 2
        duties(1) = (Tm_m1_0(1)+Tm_m1_0(3)/2);
        duties(2) = (Tm_m1_0(1)+Tm_m1_0(2)+Tm_m1_0(3)/2);
        duties(3) = (Tm_m1_0(3)/2);
    case 3
        duties(2) = (Tm_m1_0(1)+Tm_m1_0(2)+Tm_m1_0(3)/2);
        duties(3) = (Tm_m1_0(2)+Tm_m1_0(3)/2);
        duties(1) = (Tm_m1_0(3)/2);
    case 4
        duties(3) = (Tm_m1_0(1)+Tm_m1_0(2)+Tm_m1_0(3)/2);
        duties(2) = (Tm_m1_0(1)+Tm_m1_0(3)/2);
        duties(1) = (Tm_m1_0(3)/2);
    case 5
        duties(3) = (Tm_m1_0(1)+Tm_m1_0(2)+Tm_m1_0(3)/2);
        duties(1) = (Tm_m1_0(2)+Tm_m1_0(3)/2);
        duties(2) = (Tm_m1_0(3)/2);
    case 6
        duties(1) = (Tm_m1_0(1)+Tm_m1_0(2)+Tm_m1_0(3)/2);
        duties(3) = (Tm_m1_0(1)+Tm_m1_0(3)/2);
        duties(2) = (Tm_m1_0(3)/2);
end
   duties = duties./inv.Tpwm;

% calculation of uAref_sat, uBref_sat from uABref
if Tm_m1_0(3)<=0
    H = Tabc_AB0*(duties.*inv.Ubus);
    uAref_sat = [1 0 0]*H;
    uBref_sat = [0 1 0]*H;  
else
    uAref_sat = uABref(1);
    uBref_sat = uABref(2);
end

== matlab function SalientPolePMSM/FOC1/INVERTER2/SVM algorithm/MATLAB Function ==
  data: XYZ input; sector output; duty output
function [sector,duty] = sector_identifier(XYZ)
% this function find the sector in the SVM where uABref is
PWMperiod = 1/16000;

X = XYZ(1);
Y = XYZ(2);
Z = XYZ(3);

TimePhA = 0;
TimePhB = 0; 
TimePhC = 0;

if(Y < 0) 
    if(Z < 0) 
        sector = 5;
        TimePhA = (PWMperiod/2) + (Y - Z)/2;
        TimePhB = TimePhA + Z;
        TimePhC = TimePhA - Y;
    else
        if( X <= 0)
            sector = 4
            TimePhA = (PWMperiod/2) + (X - Z)/2;
            TimePhB = TimePhA + Z;
            TimePhC = TimePhB - X;
        else
            sector = 3;
            TimePhA = (PWMperiod/2) + (Y - X) /2;
            TimePhC = TimePhA - Y;
            TimePhB = TimePhC + X;
        end
    end
else
    if(Z>=0)
        sector = 2;
        TimePhA = (PWMperiod/2) + (Y - Z)/2;
        TimePhB = TimePhA + Z;
        TimePhC = TimePhA - Y;
    else
        if (X<=0)
            sector = 6;
            TimePhA = (PWMperiod/2) + (Y - X) /2;
            TimePhC = TimePhA - Y;
            TimePhB = TimePhC + X;
        else
            sector = 1;
            TimePhA = (PWMperiod/2) + (X - Z)/2;
            TimePhB = TimePhA + Z;
            TimePhC = TimePhB - X;
        end
    end
end

duty = [TimePhA*16000, TimePhB*16000, TimePhC*16000];
end

== matlab function SalientPolePMSM/FOC1/INVERTER2/SVM algorithm/MATLAB Function4 ==
  data: VABref input; X output; Y output; Z output
function [X,Y,Z] = AB2XYZ(VABref)
% this function find the sector in the SVM where uABref is

PWM_period = 1/16000;
Valpha = VABref(1);
Vbeta = VABref(2);

Ualpha = Valpha * sqrt(3) * PWM_period;
Ubeta = -(Vbeta * PWM_period);

X = Ubeta;
Y = (Ubeta + Ualpha)/2;
Z = (Ubeta - Ualpha) / 2;
end

== matlab function SalientPolePMSM/FOC1/PI_curr1/MATLAB Function1 ==
  settings: updateMethod=DISCRETE  sampleTime=inv.Ts
  data: u input; y output; inv parameter; kid parameter; kpd parameter
function y = PI_iq(u,inv, kid, kpd)
persistent err_int
if isempty(err_int)
    err_int =0;
end

kpd = 0.125;
kid = 0.00781;
y_prop = kpd*u; % P- part
err_int = err_int + kid*u; % I- part

% limit the integral
if err_int > inv.U_lim
    err_int = inv.U_lim;
end
if err_int < -inv.U_lim
    err_int = -inv.U_lim;
end

% compute the output voltage reference
y = y_prop + err_int;

% limit the PI output
if y > inv.U_lim
    y = inv.U_lim;
end
if y < -inv.U_lim
    y = -inv.U_lim;
end

end

== matlab function SalientPolePMSM/FOC1/PI_curr1/MATLAB Function3 ==
  settings: updateMethod=DISCRETE  sampleTime=inv.Ts
  data: u input; y output; inv parameter; kid parameter; kpd parameter
function y = PI_id(u,inv,kid, kpd)
persistent err_int
if isempty(err_int)
    err_int =0;
end

kpd = 0.125;
kid = 0.00781;
y_prop = kpd*u; % P- part
err_int = err_int + kid*u; % I- part

% limit the integral
if err_int > inv.U_lim
    err_int = inv.U_lim;
end
if err_int < -inv.U_lim
    err_int = -inv.U_lim;
end

% compute the output voltage reference
y = y_prop + err_int;

% limit the PI output
if y > inv.U_lim
    y = inv.U_lim;
end
if y < -inv.U_lim
    y = -inv.U_lim;
end

end

== matlab function SalientPolePMSM/FOC1/PI_curr2/MATLAB Function1 ==
  settings: updateMethod=DISCRETE  sampleTime=inv.Ts
  data: u input; y output; inv parameter; PI parameter
function y = PI_iq(u,inv,PI)
persistent err_int
if isempty(err_int)
    err_int =0;
end

kpd = PI.cur.kpd;
kid = PI.cur.kid;
y_prop = kpd*u; % P- part
err_int = err_int + kid*u; % I- part

% limit the integral
if err_int > inv.U_lim
    err_int = inv.U_lim;
end
if err_int < -inv.U_lim
    err_int = -inv.U_lim;
end

% compute the output voltage reference
y = y_prop + err_int;

% limit the PI output
if y > inv.U_lim
    y = inv.U_lim;
end
if y < -inv.U_lim
    y = -inv.U_lim;
end

end

== matlab function SalientPolePMSM/FOC1/PI_curr2/MATLAB Function3 ==
  settings: updateMethod=DISCRETE  sampleTime=inv.Ts
  data: u input; y output; inv parameter; PI parameter
function y = PI_id(u,inv,PI)
persistent err_int
if isempty(err_int)
    err_int =0;
end
kpd = PI.cur.kpd;
kid = PI.cur.kid;
y_prop = kpd*u; % P- part
err_int = err_int + kid*u; % I- part

% limit the integral
if err_int > inv.U_lim
    err_int = inv.U_lim;
end
if err_int < -inv.U_lim
    err_int = -inv.U_lim;
end

% compute the output voltage reference
y = y_prop + err_int;

%limit the PI output
if y > inv.U_lim
    y = inv.U_lim;
end
if y < -inv.U_lim
   y = -inv.U_lim;
end

end

== matlab function SalientPolePMSM/INVERTER/SVM algorithm/MATLAB Function2 ==
  data: sid input; Tm_m1_0 output; uABref input; uBus input; inv parameter
function Tm_m1_0 = application_time(sid, uABref, uBus, inv)
%this function calculate the application time Tm Tm+1 and T0

Tm_m1_0 = zeros(3,1);

    % PROBLEMA DI PASSAGGIO DELLA VARIABILE ALLA FUNZIONE

Tm_m1_0(1)=sqrt(3)/uBus*inv.Tpwm*(uABref(1)*inv.sector_LUT(sid,1)-uABref(2)*inv.sector_LUT(sid,2));
Tm_m1_0(2)=sqrt(3)/uBus*inv.Tpwm*(-uABref(1)*inv.sector_LUT(sid,3)+uABref(2)*inv.sector_LUT(sid,4));
Tm_m1_0(3)=inv.Tpwm-Tm_m1_0(1)-Tm_m1_0(2);

== matlab function SalientPolePMSM/DT SENSORLESS ALGORITHM DQ/Classic PLL1/MATLAB Function1 ==
  data: u input; y output
function y = fcn(u)

if(u < 0)
    y = u * -1;
else
    y = u;
end

== matlab function SalientPolePMSM/Discrete SS ALGORITHM/MATLAB Function3 ==
  data: u input; y output
function y = fcn(u)

if(u < 0)
    y = u * -1;
else
    y = u;
end

== matlab function SalientPolePMSM/MATLAB Function4 ==
  data: th input; thMod output
function thMod = ModulAxis(th)
% th[rad]-> 0<thMod<2*pi
n = abs(th/(2*pi));
if n>1
    if th>0
        thMod = th-floor(n)*2*pi;
    else
        thMod = th+floor(n)*2*pi;
    end
else
    thMod = th;
end

== matlab function SalientPolePMSM/MATLAB Function5 ==
  data: th input; thMod output
function thMod = ModulAxis(th)
% th[rad]-> 0<thMod<2*pi
n = abs(th/(2*pi));
if n>1
    if th>0
        thMod = th-floor(n)*2*pi;
    else
        thMod = th+floor(n)*2*pi;
    end
else
    thMod = th;
end

== matlab function SalientPolePMSM/SENSORLESS ALGORITHM1/atan ==
  data: ed input; thme output; eq input
function thme = atan(ed,eq)

thme = atan2(-ed,eq);

== matlab function SalientPolePMSM/SENSORLESS ALGORITHM1/atanApprox ==
  data: id input; ed input; thme output; wme_est input; dqpll parameter
function thme = approx(id, ed, wme_est, dqpll)
if abs(wme_est)<dqpll.minw
    wme_est = dqpll.minw;
end
Eex = wme_est*((dqpll.Ld-dqpll.Lq)*id+dqpll.lammg);
thme = -ed/Eex;

== matlab function SalientPolePMSM/SENSORLESS1 ==
  data: iabc input; thme_est output; uabc input; ON_approx input; wme_est output; dqpll parameter; data input
function [thme_est,wme_est] = dqPLL_Sensorless(iabc, uabc, ON_approx, dqpll, data)

% sensorless algorithm based on dq-PLL loop

persistent Xd_1 Xq_1 thme_est_1 wme_est_1 ui_1 Dth_1
if isempty(Xd_1)
    Xd_1 = [0 0]';
    Xq_1 = [0 0]';
    thme_est_1 = 0;
    wme_est_1 = 0;
end
if isempty(ui_1)
    ui_1 = 0;
    Dth_1 = 0;
end

% compute abc->dq transformation
iAB0 = dqpll.Tabc_AB0*iabc;
idq = zeros(1,2);
idq(1) = iAB0(1)*cos(thme_est_1)+iAB0(2)*sin(thme_est_1);
idq(2) = -iAB0(1)*sin(thme_est_1)+iAB0(2)*cos(thme_est_1);

uAB0 = dqpll.Tabc_AB0*uabc;
udq = zeros(1,2);
udq(1) = uAB0(1)*cos(thme_est_1)+uAB0(2)*sin(thme_est_1);
udq(2) = -uAB0(1)*sin(thme_est_1)+uAB0(2)*cos(thme_est_1);

% DECOUPLING for ud and uq
udq(1) = udq(1) + wme_est_1*idq(2)*dqpll.Lq;
udq(2) = udq(2) - wme_est_1*idq(1)*dqpll.Lq;

% ESTIMATOR of ed and eq
Xd = dqpll.est.F1*Xd_1 + dqpll.est.G1*[udq(1) idq(1)]';
Xq = dqpll.est.F1*Xq_1 + dqpll.est.G1*[udq(2) idq(2)]';
ed = dqpll.est.H1*Xd;
eq = dqpll.est.H1*Xq;

% atan calculation
if ON_approx == 0
    Dth = atan2(-ed,eq);
else
    if abs(wme_est_1)<dqpll.minw
        w = dqpll.minw;
    else
        w = wme_est_1;
    end
    Eex = w*((dqpll.Ld-dqpll.Lq)*idq(1)+dqpll.lammg);
    Dth = -ed/Eex;
end

% PI loop
up = Dth*dqpll.PI.kp;
ui = ui_1 + Dth_1*dqpll.Ts;
wme = up + ui*dqpll.PI.ki;

% calculation of thme with EULER INTEGRATION
thme_est = thme_est_1 + dqpll.Ts*wme;

% Low Pass Filter for wme_est
wme_est = dqpll.lpf.alpha*wme + (1-dqpll.lpf.alpha)*wme_est_1;

% update variables
thme_est_1 = thme_est;
wme_est_1 = wme_est;
ui_1 = ui;
Dth_1 = Dth;
Xd_1 = Xd;
Xq_1 = Xq;
